simulink model "IP_Core_SS_Switch_and_PWM"  (R2021a)
settings: Solver=VariableStepAuto  StartTime=0.0  StopTime=0.001  RelTol=1e-3
values from neighbouring files (symbols this model uses):
  f_FPGA_clk = 100e6    (= 100000000)    [Init_IP_Core.m]
  T_FPGA_clk = 1/f_FPGA_clk    (= 1e-08)    [Init_IP_Core.m]
libraries: hdlsllib x4, simulink x2
(part 2 of 3)

== system IP_Core_SS_Switch_and_PWM/PWM_and_Switching_Signal_Control/GenPWM/LimitPulseWidth2 ==
  note: Set pulse width in percent
  ref_sig : Inport
  min_pulse_width : Inport  Port=2
  Add : Sum  Inputs=+-  OutDataTypeStr=Inherit: Same as first input
  Constant : Constant  OutDataTypeStr=fixdt(1,18,16)  SampleTime=T_FPGA_clk
  Constant1 : Constant  Value=1.01  OutDataTypeStr=fixdt(1,18,16)  SampleTime=T_FPGA_clk
  Constant2 : Constant  Value=0  OutDataTypeStr=fixdt(1,18,16)  SampleTime=T_FPGA_clk
  Logical Operator : Logic  Operator=OR  AllPortsSameDT=off  OutDataTypeStr=boolean
  Relational Operator : RelationalOperator  Operator=>  OutDataTypeStr=boolean  RndMeth=Nearest
  Relational Operator1 : RelationalOperator  Operator=<  OutDataTypeStr=boolean  RndMeth=Nearest
  Saturation : Saturate  UpperLimit=1  LowerLimit=0  OutDataTypeStr=fixdt(1,18,16)
  Switch1 : Switch  Criteria=u2 > Threshold
  Switch6 : Switch  Criteria=u2 > Threshold
  ref_sig_limit : Outport  VectorParamsAs1DForOutWhenUnconnected=off
  wires:
  Constant/1 -> Add/1
  min_pulse_width/1 -> Add/2, Saturation/1
  Add/1 -> Relational Operator/2
  ref_sig/1 -> Switch6/3, Relational Operator/1, Relational Operator1/1
  Relational Operator/1 -> Logical Operator/1
  Relational Operator1/1 -> Logical Operator/2, Switch1/2
  Logical Operator/1 -> Switch6/2
  Constant1/1 -> Switch1/3
  Switch1/1 -> Switch6/1
  Constant2/1 -> Switch1/1
  Switch6/1 -> ref_sig_limit/1
  Saturation/1 -> Relational Operator1/2

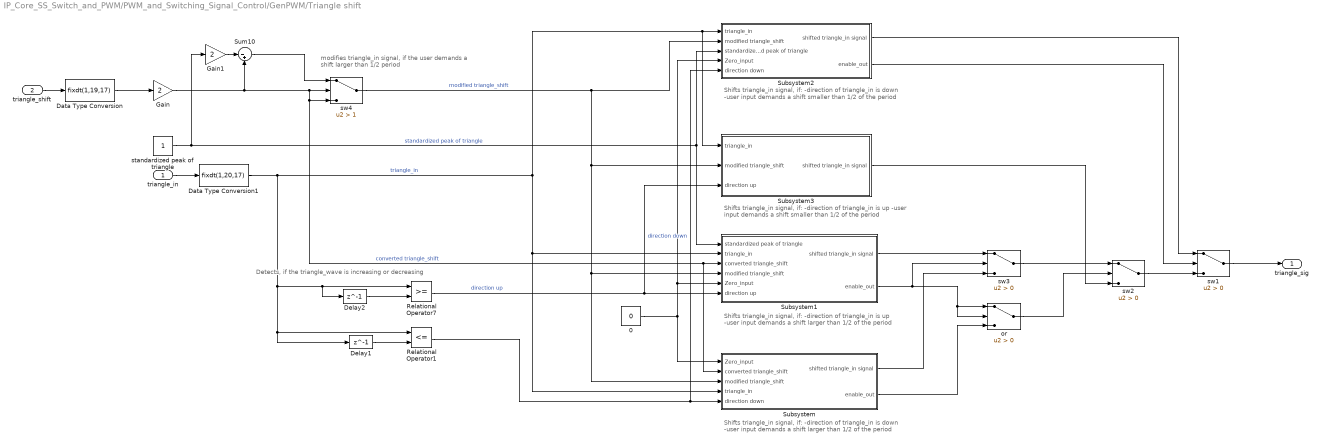
== system IP_Core_SS_Switch_and_PWM/PWM_and_Switching_Signal_Control/GenPWM/Triangle shift ==
  note: modifies triangle_in signal,
      | if the user demands a shift larger than 1/2 period
  note: Detects, if the triangle_wave is increasing or decreasing
  note: Shifts triangle_in signal, if:
      | -direction of triangle_in is down
      | -user input demands a shift larger than 1/2 of the period
  note: Shifts triangle_in signal, if:
      | -direction of triangle_in is up
      | -user input demands a shift larger than 1/2 of the period
  note: Shifts triangle_in signal, if:
      | -direction of triangle_in is up
      | -user input demands a shift smaller than 1/2 of the period
  note: Shifts triangle_in signal, if:
      | -direction of triangle_in is down
      | -user input demands a shift smaller than 1/2 of the period
  triangle_in : Inport
  triangle_shift : Inport  Port=2
  0 : Constant  Value=0  OutDataTypeStr=boolean  SampleTime=T_FPGA_clk
  Data Type Conversion : DataTypeConversion  OutDataTypeStr=fixdt(1,19,17)
  Data Type Conversion1 : DataTypeConversion  OutDataTypeStr=fixdt(1,20,17)
  Delay1 : Delay  DelayLength=1
  Delay2 : Delay  DelayLength=1
  Gain : Gain  Gain=2  OutDataTypeStr=fixdt(1,20,17)
  Gain1 : Gain  Gain=2  OutDataTypeStr=fixdt(1,20,17)
  Relational Operator1 : RelationalOperator  Operator=<=  OutDataTypeStr=boolean  RndMeth=Nearest
  Relational Operator7 : RelationalOperator  OutDataTypeStr=boolean  RndMeth=Nearest
  Subsystem : Subsystem
  Subsystem1 : Subsystem
  Subsystem2 : Subsystem
  Subsystem3 : Subsystem
  Sum10 : Sum  Inputs=|-+  OutDataTypeStr=fixdt(1,20,17)
  or : Switch  Criteria=u2 > Threshold
  standardized peak of triangle : Constant  OutDataTypeStr=fixdt(0,21,17)  SampleTime=T_FPGA_clk
  sw1 : Switch  Criteria=u2 > Threshold  OutDataTypeStr=fixdt(1,18,16)
  sw2 : Switch  Criteria=u2 > Threshold
  sw3 : Switch  Criteria=u2 > Threshold
  sw4 : Switch  Criteria=u2 > Threshold  Threshold=1  OutDataTypeStr=fixdt(1,20,17)
  triangle_sig : Outport  VectorParamsAs1DForOutWhenUnconnected=off
  wires:
  Delay2/1 -> Relational Operator7/2
  Data Type Conversion1/1 -> Subsystem3/1(triangle_in), Subsystem2/1(triangle_in), Subsystem/4(triangle_in), Subsystem1/2(triangle_in), Relational Operator1/1, Delay1/1, Delay2/1, Relational Operator7/1  "triangle_in"
  sw3/1 -> sw2/1
  Relational Operator7/1 -> Subsystem1/6(direction up), Subsystem3/3(direction up)  "direction up"
  or/1 -> sw2/2
  sw4/1 -> Subsystem3/2(modified triangle_shift), Subsystem/3(modified triangle_shift), Subsystem1/4(modified triangle_shift), Subsystem2/2(modified triangle_shift)  "modified triangle_shift"
  Gain/1 -> Sum10/2, Subsystem/2(converted triangle_shift), Subsystem1/3(converted triangle_shift), sw4/3, sw4/2  "converted triangle_shift"
  Sum10/1 -> sw4/1
  sw1/1 -> triangle_sig/1
  standardized peak of triangle/1 -> Subsystem2/3(standardized peak of triangle), Subsystem1/1(standardized peak of triangle), Gain1/1  "standardized peak of triangle"
  triangle_shift/1 -> Data Type Conversion/1
  Gain1/1 -> Sum10/1
  sw2/1 -> sw1/3
  Data Type Conversion/1 -> Gain/1
  triangle_in/1 -> Data Type Conversion1/1
  Relational Operator1/1 -> Subsystem/5(direction down), Subsystem2/5(direction down)  "direction down"
  Delay1/1 -> Relational Operator1/2
  0/1 -> Subsystem2/4(Zero_input), Subsystem1/5(Zero_input), Subsystem/1(Zero_input)
  Subsystem/1(shifted triangle_in signal) -> sw3/3
  Subsystem/2(enable_out) -> or/3
  Subsystem1/2(enable_out) -> or/2, or/1, sw3/2
  Subsystem1/1(shifted triangle_in signal) -> sw3/1
  Subsystem2/1(shifted triangle_in signal) -> sw1/1
  Subsystem2/2(enable_out) -> sw1/2
  Subsystem3/1(shifted triangle_in signal) -> sw2/3

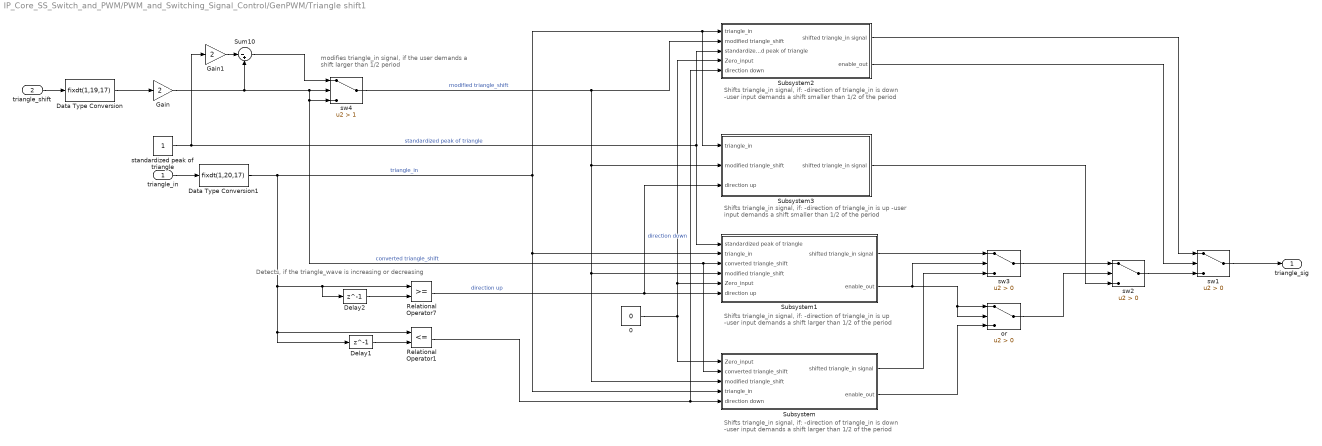
== system IP_Core_SS_Switch_and_PWM/PWM_and_Switching_Signal_Control/GenPWM/Triangle shift1 ==
  note: modifies triangle_in signal,
      | if the user demands a shift larger than 1/2 period
  note: Detects, if the triangle_wave is increasing or decreasing
  note: Shifts triangle_in signal, if:
      | -direction of triangle_in is down
      | -user input demands a shift larger than 1/2 of the period
  note: Shifts triangle_in signal, if:
      | -direction of triangle_in is up
      | -user input demands a shift larger than 1/2 of the period
  note: Shifts triangle_in signal, if:
      | -direction of triangle_in is up
      | -user input demands a shift smaller than 1/2 of the period
  note: Shifts triangle_in signal, if:
      | -direction of triangle_in is down
      | -user input demands a shift smaller than 1/2 of the period
  triangle_in : Inport
  triangle_shift : Inport  Port=2
  0 : Constant  Value=0  OutDataTypeStr=boolean  SampleTime=T_FPGA_clk
  Data Type Conversion : DataTypeConversion  OutDataTypeStr=fixdt(1,19,17)
  Data Type Conversion1 : DataTypeConversion  OutDataTypeStr=fixdt(1,20,17)
  Delay1 : Delay  DelayLength=1
  Delay2 : Delay  DelayLength=1
  Gain : Gain  Gain=2  OutDataTypeStr=fixdt(1,20,17)
  Gain1 : Gain  Gain=2  OutDataTypeStr=fixdt(1,20,17)
  Relational Operator1 : RelationalOperator  Operator=<=  OutDataTypeStr=boolean  RndMeth=Nearest
  Relational Operator7 : RelationalOperator  OutDataTypeStr=boolean  RndMeth=Nearest
  Subsystem : Subsystem
  Subsystem1 : Subsystem
  Subsystem2 : Subsystem
  Subsystem3 : Subsystem
  Sum10 : Sum  Inputs=|-+  OutDataTypeStr=fixdt(1,20,17)
  or : Switch  Criteria=u2 > Threshold
  standardized peak of triangle : Constant  OutDataTypeStr=fixdt(0,21,17)  SampleTime=T_FPGA_clk
  sw1 : Switch  Criteria=u2 > Threshold  OutDataTypeStr=fixdt(1,18,16)
  sw2 : Switch  Criteria=u2 > Threshold
  sw3 : Switch  Criteria=u2 > Threshold
  sw4 : Switch  Criteria=u2 > Threshold  Threshold=1  OutDataTypeStr=fixdt(1,20,17)
  triangle_sig : Outport  VectorParamsAs1DForOutWhenUnconnected=off
  wires:
  Delay2/1 -> Relational Operator7/2
  Data Type Conversion1/1 -> Subsystem3/1(triangle_in), Subsystem2/1(triangle_in), Subsystem/4(triangle_in), Subsystem1/2(triangle_in), Relational Operator1/1, Delay1/1, Delay2/1, Relational Operator7/1  "triangle_in"
  sw3/1 -> sw2/1
  Relational Operator7/1 -> Subsystem1/6(direction up), Subsystem3/3(direction up)  "direction up"
  or/1 -> sw2/2
  sw4/1 -> Subsystem3/2(modified triangle_shift), Subsystem/3(modified triangle_shift), Subsystem1/4(modified triangle_shift), Subsystem2/2(modified triangle_shift)  "modified triangle_shift"
  Gain/1 -> Sum10/2, Subsystem/2(converted triangle_shift), Subsystem1/3(converted triangle_shift), sw4/3, sw4/2  "converted triangle_shift"
  Sum10/1 -> sw4/1
  sw1/1 -> triangle_sig/1
  standardized peak of triangle/1 -> Subsystem2/3(standardized peak of triangle), Subsystem1/1(standardized peak of triangle), Gain1/1  "standardized peak of triangle"
  triangle_shift/1 -> Data Type Conversion/1
  Gain1/1 -> Sum10/1
  sw2/1 -> sw1/3
  Data Type Conversion/1 -> Gain/1
  triangle_in/1 -> Data Type Conversion1/1
  Relational Operator1/1 -> Subsystem/5(direction down), Subsystem2/5(direction down)  "direction down"
  Delay1/1 -> Relational Operator1/2
  0/1 -> Subsystem2/4(Zero_input), Subsystem1/5(Zero_input), Subsystem/1(Zero_input)
  Subsystem/1(shifted triangle_in signal) -> sw3/3
  Subsystem/2(enable_out) -> or/3
  Subsystem1/2(enable_out) -> or/2, or/1, sw3/2
  Subsystem1/1(shifted triangle_in signal) -> sw3/1
  Subsystem2/1(shifted triangle_in signal) -> sw1/1
  Subsystem2/2(enable_out) -> sw1/2
  Subsystem3/1(shifted triangle_in signal) -> sw2/3

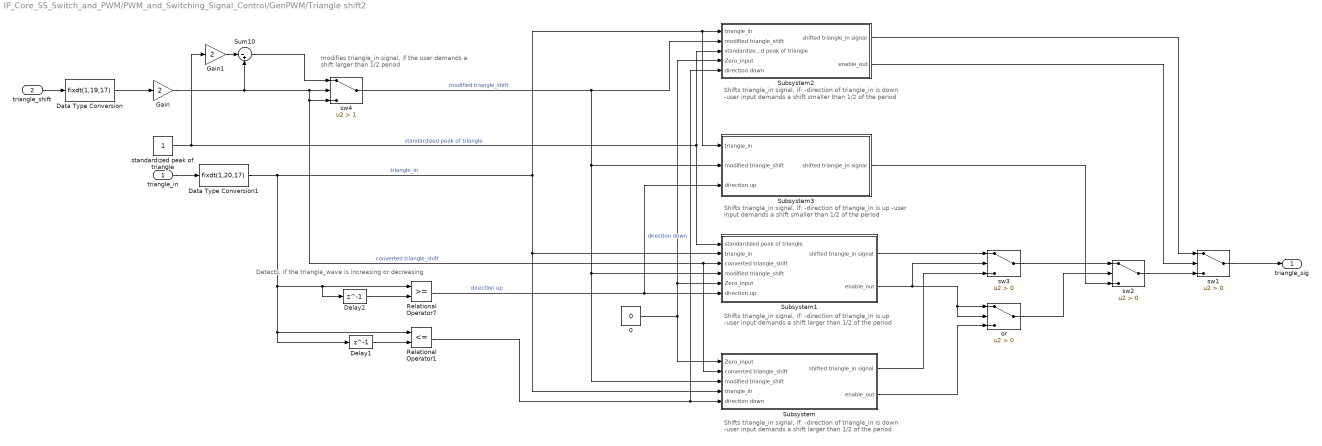
== system IP_Core_SS_Switch_and_PWM/PWM_and_Switching_Signal_Control/GenPWM/Triangle shift2 ==
  note: modifies triangle_in signal,
      | if the user demands a shift larger than 1/2 period
  note: Detects, if the triangle_wave is increasing or decreasing
  note: Shifts triangle_in signal, if:
      | -direction of triangle_in is down
      | -user input demands a shift larger than 1/2 of the period
  note: Shifts triangle_in signal, if:
      | -direction of triangle_in is up
      | -user input demands a shift larger than 1/2 of the period
  note: Shifts triangle_in signal, if:
      | -direction of triangle_in is up
      | -user input demands a shift smaller than 1/2 of the period
  note: Shifts triangle_in signal, if:
      | -direction of triangle_in is down
      | -user input demands a shift smaller than 1/2 of the period
  triangle_in : Inport
  triangle_shift : Inport  Port=2
  0 : Constant  Value=0  OutDataTypeStr=boolean  SampleTime=T_FPGA_clk
  Data Type Conversion : DataTypeConversion  OutDataTypeStr=fixdt(1,19,17)
  Data Type Conversion1 : DataTypeConversion  OutDataTypeStr=fixdt(1,20,17)
  Delay1 : Delay  DelayLength=1
  Delay2 : Delay  DelayLength=1
  Gain : Gain  Gain=2  OutDataTypeStr=fixdt(1,20,17)
  Gain1 : Gain  Gain=2  OutDataTypeStr=fixdt(1,20,17)
  Relational Operator1 : RelationalOperator  Operator=<=  OutDataTypeStr=boolean  RndMeth=Nearest
  Relational Operator7 : RelationalOperator  OutDataTypeStr=boolean  RndMeth=Nearest
  Subsystem : Subsystem
  Subsystem1 : Subsystem
  Subsystem2 : Subsystem
  Subsystem3 : Subsystem
  Sum10 : Sum  Inputs=|-+  OutDataTypeStr=fixdt(1,20,17)
  or : Switch  Criteria=u2 > Threshold
  standardized peak of triangle : Constant  OutDataTypeStr=fixdt(0,21,17)  SampleTime=T_FPGA_clk
  sw1 : Switch  Criteria=u2 > Threshold  OutDataTypeStr=fixdt(1,18,16)
  sw2 : Switch  Criteria=u2 > Threshold
  sw3 : Switch  Criteria=u2 > Threshold
  sw4 : Switch  Criteria=u2 > Threshold  Threshold=1  OutDataTypeStr=fixdt(1,20,17)
  triangle_sig : Outport  VectorParamsAs1DForOutWhenUnconnected=off
  wires:
  Delay2/1 -> Relational Operator7/2
  Data Type Conversion1/1 -> Subsystem3/1(triangle_in), Subsystem2/1(triangle_in), Subsystem/4(triangle_in), Subsystem1/2(triangle_in), Relational Operator1/1, Delay1/1, Delay2/1, Relational Operator7/1  "triangle_in"
  sw3/1 -> sw2/1
  Relational Operator7/1 -> Subsystem1/6(direction up), Subsystem3/3(direction up)  "direction up"
  or/1 -> sw2/2
  sw4/1 -> Subsystem3/2(modified triangle_shift), Subsystem/3(modified triangle_shift), Subsystem1/4(modified triangle_shift), Subsystem2/2(modified triangle_shift)  "modified triangle_shift"
  Gain/1 -> Sum10/2, Subsystem/2(converted triangle_shift), Subsystem1/3(converted triangle_shift), sw4/3, sw4/2  "converted triangle_shift"
  Sum10/1 -> sw4/1
  sw1/1 -> triangle_sig/1
  standardized peak of triangle/1 -> Subsystem2/3(standardized peak of triangle), Subsystem1/1(standardized peak of triangle), Gain1/1  "standardized peak of triangle"
  triangle_shift/1 -> Data Type Conversion/1
  Gain1/1 -> Sum10/1
  sw2/1 -> sw1/3
  Data Type Conversion/1 -> Gain/1
  triangle_in/1 -> Data Type Conversion1/1
  Relational Operator1/1 -> Subsystem/5(direction down), Subsystem2/5(direction down)  "direction down"
  Delay1/1 -> Relational Operator1/2
  0/1 -> Subsystem2/4(Zero_input), Subsystem1/5(Zero_input), Subsystem/1(Zero_input)
  Subsystem/1(shifted triangle_in signal) -> sw3/3
  Subsystem/2(enable_out) -> or/3
  Subsystem1/2(enable_out) -> or/2, or/1, sw3/2
  Subsystem1/1(shifted triangle_in signal) -> sw3/1
  Subsystem2/1(shifted triangle_in signal) -> sw1/1
  Subsystem2/2(enable_out) -> sw1/2
  Subsystem3/1(shifted triangle_in signal) -> sw2/3

== system IP_Core_SS_Switch_and_PWM/PWM_and_Switching_Signal_Control1/GenPWM/Counter Ctrl ==
  note: if (hdl_cnt >= step_cnt)
      | 	dir_ctrl = true;
      | else if (hdl_cnt <= 0)
      | 	dir_ctrl = false;
      | else
      | 	dir_ctrl = dir_ctrl;
  note: scaling triangle amplitude to 100
  hdl_cnt : Inport
  f_carrier_kHz : Inport  Port=2
  T_carrier_us : Inport  Port=3
  Constant1 : Constant  Value=0  OutDataTypeStr=fixdt(0,20,0)  SampleTime=T_FPGA_clk
  Constant11 : Constant  Value=0  OutDataTypeStr=fixdt(0,20,0)  SampleTime=T_FPGA_clk
  Constant12 : Constant  Value=false  SampleTime=T_FPGA_clk
  Constant14 : Constant  Value=true  SampleTime=T_FPGA_clk
  Delay : Delay  DelayLength=1
  Delay6 : Delay  DelayLength=1
  Logical Operator : Logic  Operator=OR  AllPortsSameDT=off  OutDataTypeStr=boolean
  Product : Product  OutDataTypeStr=fixdt(0,18,17)
  Relational Operator1 : RelationalOperator  Operator===  OutDataTypeStr=boolean  RndMeth=Nearest
  Relational Operator2 : RelationalOperator  Operator===  OutDataTypeStr=boolean  RndMeth=Nearest
  Relational Operator4 : RelationalOperator  OutDataTypeStr=boolean  RndMeth=Nearest
  Relational Operator5 : RelationalOperator  Operator=<=  OutDataTypeStr=boolean  RndMeth=Nearest
  Scope9 : Scope  NumInputPorts=2
  Switch6 : Switch  Criteria=u2 > Threshold
  Switch7 : Switch  Criteria=u2 > Threshold
  dir_ctrl : Outport  VectorParamsAs1DForOutWhenUnconnected=off
  triangle_sig : Outport  Port=2  VectorParamsAs1DForOutWhenUnconnected=off
  Period_CenterMax : Outport  Port=3  VectorParamsAs1DForOutWhenUnconnected=off
  Period_CenterMin : Outport  Port=4  VectorParamsAs1DForOutWhenUnconnected=off
  wires:
  hdl_cnt/1 -> Relational Operator2/1, Relational Operator1/1, Relational Operator5/1, Relational Operator4/1, Product/1, Scope9/1
  Switch6/1 -> Delay6/1, dir_ctrl/1
  Relational Operator4/1 -> Switch7/2, Logical Operator/1
  Relational Operator5/1 -> Logical Operator/2
  Constant11/1 -> Relational Operator5/2
  Logical Operator/1 -> Switch6/2
  Switch7/1 -> Switch6/1
  Constant12/1 -> Switch7/1
  Constant14/1 -> Switch7/3
  Delay6/1 -> Switch6/3
  T_carrier_us/1 -> Relational Operator4/2, Relational Operator1/2
  f_carrier_kHz/1 -> Delay/1
  Delay/1 -> Scope9/2, Product/2
  Relational Operator1/1 -> Period_CenterMax/1
  Relational Operator2/1 -> Period_CenterMin/1
  Constant1/1 -> Relational Operator2/2
  Product/1 -> triangle_sig/1

== system IP_Core_SS_Switch_and_PWM/PWM_and_Switching_Signal_Control1/GenPWM/LimitPulseWidth ==
  note: Set pulse width between 0-1
  ref_sig : Inport
  min_pulse_width : Inport  Port=2
  Add : Sum  Inputs=+-  OutDataTypeStr=Inherit: Same as first input
  Constant : Constant  OutDataTypeStr=fixdt(1,18,16)  SampleTime=T_FPGA_clk
  Constant1 : Constant  Value=1.01  OutDataTypeStr=fixdt(1,18,16)  SampleTime=T_FPGA_clk
  Constant2 : Constant  Value=0  OutDataTypeStr=fixdt(1,18,16)  SampleTime=T_FPGA_clk
  Logical Operator : Logic  Operator=OR  AllPortsSameDT=off  OutDataTypeStr=boolean
  Relational Operator : RelationalOperator  Operator=>  OutDataTypeStr=boolean  RndMeth=Nearest
  Relational Operator1 : RelationalOperator  Operator=<  OutDataTypeStr=boolean  RndMeth=Nearest
  Saturation : Saturate  UpperLimit=1  LowerLimit=0  OutDataTypeStr=fixdt(1,18,16)
  Switch1 : Switch  Criteria=u2 > Threshold
  Switch6 : Switch  Criteria=u2 > Threshold
  ref_sig_limit : Outport  VectorParamsAs1DForOutWhenUnconnected=off
  wires:
  Constant/1 -> Add/1
  min_pulse_width/1 -> Add/2, Saturation/1
  Add/1 -> Relational Operator/2
  ref_sig/1 -> Switch6/3, Relational Operator/1, Relational Operator1/1
  Relational Operator/1 -> Logical Operator/1
  Relational Operator1/1 -> Logical Operator/2, Switch1/2
  Logical Operator/1 -> Switch6/2
  Constant1/1 -> Switch1/3
  Switch1/1 -> Switch6/1
  Constant2/1 -> Switch1/1
  Switch6/1 -> ref_sig_limit/1
  Saturation/1 -> Relational Operator1/2

== system IP_Core_SS_Switch_and_PWM/PWM_and_Switching_Signal_Control1/GenPWM/LimitPulseWidth1 ==
  note: Set pulse width in percent
  ref_sig : Inport
  min_pulse_width : Inport  Port=2
  Add : Sum  Inputs=+-  OutDataTypeStr=Inherit: Same as first input
  Constant : Constant  OutDataTypeStr=fixdt(1,18,16)  SampleTime=T_FPGA_clk
  Constant1 : Constant  Value=1.01  OutDataTypeStr=fixdt(1,18,16)  SampleTime=T_FPGA_clk
  Constant2 : Constant  Value=0  OutDataTypeStr=fixdt(1,18,16)  SampleTime=T_FPGA_clk
  Logical Operator : Logic  Operator=OR  AllPortsSameDT=off  OutDataTypeStr=boolean
  Relational Operator : RelationalOperator  Operator=>  OutDataTypeStr=boolean  RndMeth=Nearest
  Relational Operator1 : RelationalOperator  Operator=<  OutDataTypeStr=boolean  RndMeth=Nearest
  Saturation : Saturate  UpperLimit=1  LowerLimit=0  OutDataTypeStr=fixdt(1,18,16)
  Switch1 : Switch  Criteria=u2 > Threshold
  Switch6 : Switch  Criteria=u2 > Threshold
  ref_sig_limit : Outport  VectorParamsAs1DForOutWhenUnconnected=off
  wires:
  Constant/1 -> Add/1
  min_pulse_width/1 -> Add/2, Saturation/1
  Add/1 -> Relational Operator/2
  ref_sig/1 -> Switch6/3, Relational Operator/1, Relational Operator1/1
  Relational Operator/1 -> Logical Operator/1
  Relational Operator1/1 -> Logical Operator/2, Switch1/2
  Logical Operator/1 -> Switch6/2
  Constant1/1 -> Switch1/3
  Switch1/1 -> Switch6/1
  Constant2/1 -> Switch1/1
  Switch6/1 -> ref_sig_limit/1
  Saturation/1 -> Relational Operator1/2

== system IP_Core_SS_Switch_and_PWM/PWM_and_Switching_Signal_Control1/GenPWM/LimitPulseWidth2 ==
  note: Set pulse width in percent
  ref_sig : Inport
  min_pulse_width : Inport  Port=2
  Add : Sum  Inputs=+-  OutDataTypeStr=Inherit: Same as first input
  Constant : Constant  OutDataTypeStr=fixdt(1,18,16)  SampleTime=T_FPGA_clk
  Constant1 : Constant  Value=1.01  OutDataTypeStr=fixdt(1,18,16)  SampleTime=T_FPGA_clk
  Constant2 : Constant  Value=0  OutDataTypeStr=fixdt(1,18,16)  SampleTime=T_FPGA_clk
  Logical Operator : Logic  Operator=OR  AllPortsSameDT=off  OutDataTypeStr=boolean
  Relational Operator : RelationalOperator  Operator=>  OutDataTypeStr=boolean  RndMeth=Nearest
  Relational Operator1 : RelationalOperator  Operator=<  OutDataTypeStr=boolean  RndMeth=Nearest
  Saturation : Saturate  UpperLimit=1  LowerLimit=0  OutDataTypeStr=fixdt(1,18,16)
  Switch1 : Switch  Criteria=u2 > Threshold
  Switch6 : Switch  Criteria=u2 > Threshold
  ref_sig_limit : Outport  VectorParamsAs1DForOutWhenUnconnected=off
  wires:
  Constant/1 -> Add/1
  min_pulse_width/1 -> Add/2, Saturation/1
  Add/1 -> Relational Operator/2
  ref_sig/1 -> Switch6/3, Relational Operator/1, Relational Operator1/1
  Relational Operator/1 -> Logical Operator/1
  Relational Operator1/1 -> Logical Operator/2, Switch1/2
  Logical Operator/1 -> Switch6/2
  Constant1/1 -> Switch1/3
  Switch1/1 -> Switch6/1
  Constant2/1 -> Switch1/1
  Switch6/1 -> ref_sig_limit/1
  Saturation/1 -> Relational Operator1/2

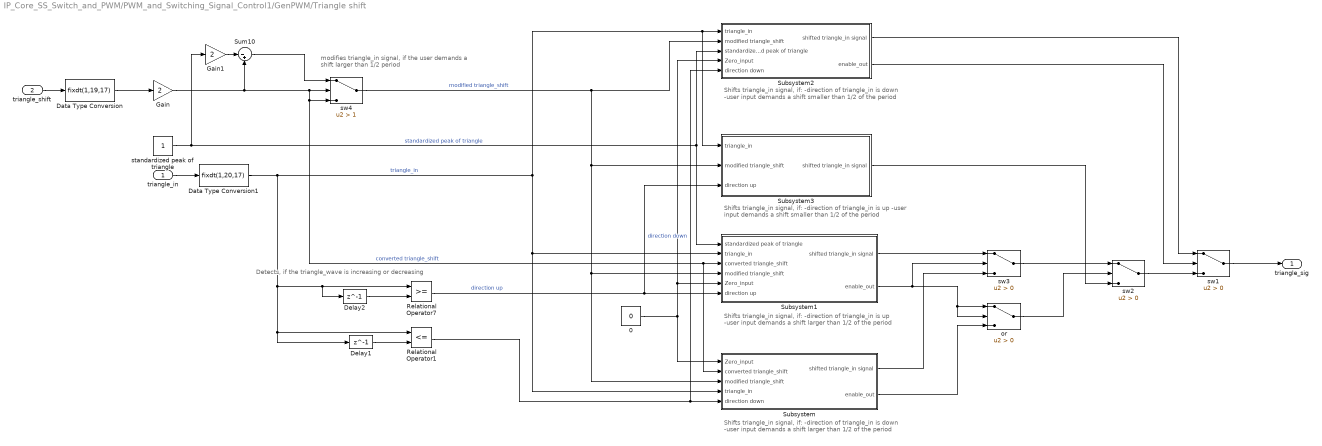
== system IP_Core_SS_Switch_and_PWM/PWM_and_Switching_Signal_Control1/GenPWM/Triangle shift ==
  note: modifies triangle_in signal,
      | if the user demands a shift larger than 1/2 period
  note: Detects, if the triangle_wave is increasing or decreasing
  note: Shifts triangle_in signal, if:
      | -direction of triangle_in is down
      | -user input demands a shift larger than 1/2 of the period
  note: Shifts triangle_in signal, if:
      | -direction of triangle_in is up
      | -user input demands a shift larger than 1/2 of the period
  note: Shifts triangle_in signal, if:
      | -direction of triangle_in is up
      | -user input demands a shift smaller than 1/2 of the period
  note: Shifts triangle_in signal, if:
      | -direction of triangle_in is down
      | -user input demands a shift smaller than 1/2 of the period
  triangle_in : Inport
  triangle_shift : Inport  Port=2
  0 : Constant  Value=0  OutDataTypeStr=boolean  SampleTime=T_FPGA_clk
  Data Type Conversion : DataTypeConversion  OutDataTypeStr=fixdt(1,19,17)
  Data Type Conversion1 : DataTypeConversion  OutDataTypeStr=fixdt(1,20,17)
  Delay1 : Delay  DelayLength=1
  Delay2 : Delay  DelayLength=1
  Gain : Gain  Gain=2  OutDataTypeStr=fixdt(1,20,17)
  Gain1 : Gain  Gain=2  OutDataTypeStr=fixdt(1,20,17)
  Relational Operator1 : RelationalOperator  Operator=<=  OutDataTypeStr=boolean  RndMeth=Nearest
  Relational Operator7 : RelationalOperator  OutDataTypeStr=boolean  RndMeth=Nearest
  Subsystem : Subsystem
  Subsystem1 : Subsystem
  Subsystem2 : Subsystem
  Subsystem3 : Subsystem
  Sum10 : Sum  Inputs=|-+  OutDataTypeStr=fixdt(1,20,17)
  or : Switch  Criteria=u2 > Threshold
  standardized peak of triangle : Constant  OutDataTypeStr=fixdt(0,21,17)  SampleTime=T_FPGA_clk
  sw1 : Switch  Criteria=u2 > Threshold  OutDataTypeStr=fixdt(1,18,16)
  sw2 : Switch  Criteria=u2 > Threshold
  sw3 : Switch  Criteria=u2 > Threshold
  sw4 : Switch  Criteria=u2 > Threshold  Threshold=1  OutDataTypeStr=fixdt(1,20,17)
  triangle_sig : Outport  VectorParamsAs1DForOutWhenUnconnected=off
  wires:
  Delay2/1 -> Relational Operator7/2
  Data Type Conversion1/1 -> Subsystem3/1(triangle_in), Subsystem2/1(triangle_in), Subsystem/4(triangle_in), Subsystem1/2(triangle_in), Relational Operator1/1, Delay1/1, Delay2/1, Relational Operator7/1  "triangle_in"
  sw3/1 -> sw2/1
  Relational Operator7/1 -> Subsystem1/6(direction up), Subsystem3/3(direction up)  "direction up"
  or/1 -> sw2/2
  sw4/1 -> Subsystem3/2(modified triangle_shift), Subsystem/3(modified triangle_shift), Subsystem1/4(modified triangle_shift), Subsystem2/2(modified triangle_shift)  "modified triangle_shift"
  Gain/1 -> Sum10/2, Subsystem/2(converted triangle_shift), Subsystem1/3(converted triangle_shift), sw4/3, sw4/2  "converted triangle_shift"
  Sum10/1 -> sw4/1
  sw1/1 -> triangle_sig/1
  standardized peak of triangle/1 -> Subsystem2/3(standardized peak of triangle), Subsystem1/1(standardized peak of triangle), Gain1/1  "standardized peak of triangle"
  triangle_shift/1 -> Data Type Conversion/1
  Gain1/1 -> Sum10/1
  sw2/1 -> sw1/3
  Data Type Conversion/1 -> Gain/1
  triangle_in/1 -> Data Type Conversion1/1
  Relational Operator1/1 -> Subsystem/5(direction down), Subsystem2/5(direction down)  "direction down"
  Delay1/1 -> Relational Operator1/2
  0/1 -> Subsystem2/4(Zero_input), Subsystem1/5(Zero_input), Subsystem/1(Zero_input)
  Subsystem/1(shifted triangle_in signal) -> sw3/3
  Subsystem/2(enable_out) -> or/3
  Subsystem1/2(enable_out) -> or/2, or/1, sw3/2
  Subsystem1/1(shifted triangle_in signal) -> sw3/1
  Subsystem2/1(shifted triangle_in signal) -> sw1/1
  Subsystem2/2(enable_out) -> sw1/2
  Subsystem3/1(shifted triangle_in signal) -> sw2/3

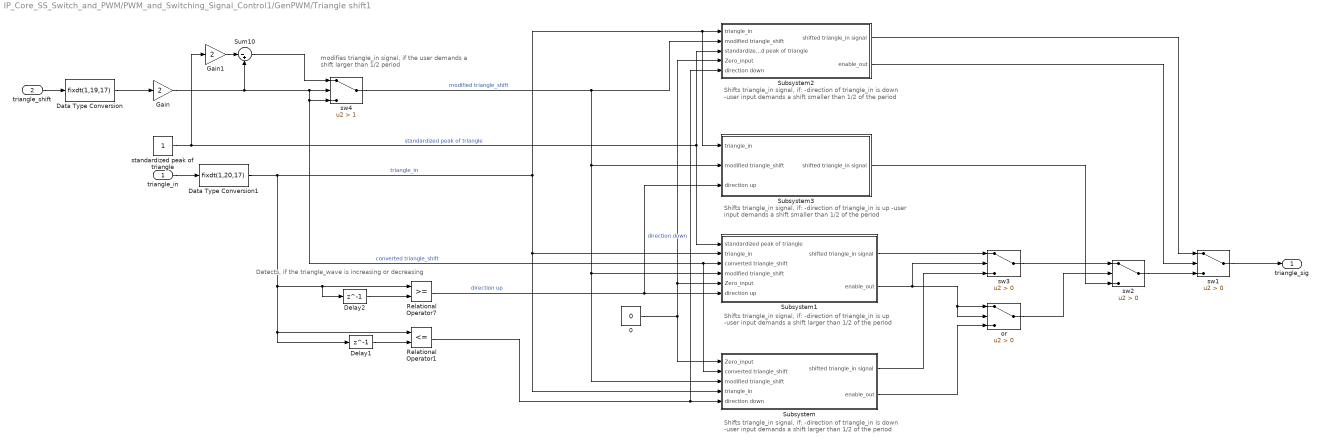
== system IP_Core_SS_Switch_and_PWM/PWM_and_Switching_Signal_Control1/GenPWM/Triangle shift1 ==
  note: modifies triangle_in signal,
      | if the user demands a shift larger than 1/2 period
  note: Detects, if the triangle_wave is increasing or decreasing
  note: Shifts triangle_in signal, if:
      | -direction of triangle_in is down
      | -user input demands a shift larger than 1/2 of the period
  note: Shifts triangle_in signal, if:
      | -direction of triangle_in is up
      | -user input demands a shift larger than 1/2 of the period
  note: Shifts triangle_in signal, if:
      | -direction of triangle_in is up
      | -user input demands a shift smaller than 1/2 of the period
  note: Shifts triangle_in signal, if:
      | -direction of triangle_in is down
      | -user input demands a shift smaller than 1/2 of the period
  triangle_in : Inport
  triangle_shift : Inport  Port=2
  0 : Constant  Value=0  OutDataTypeStr=boolean  SampleTime=T_FPGA_clk
  Data Type Conversion : DataTypeConversion  OutDataTypeStr=fixdt(1,19,17)
  Data Type Conversion1 : DataTypeConversion  OutDataTypeStr=fixdt(1,20,17)
  Delay1 : Delay  DelayLength=1
  Delay2 : Delay  DelayLength=1
  Gain : Gain  Gain=2  OutDataTypeStr=fixdt(1,20,17)
  Gain1 : Gain  Gain=2  OutDataTypeStr=fixdt(1,20,17)
  Relational Operator1 : RelationalOperator  Operator=<=  OutDataTypeStr=boolean  RndMeth=Nearest
  Relational Operator7 : RelationalOperator  OutDataTypeStr=boolean  RndMeth=Nearest
  Subsystem : Subsystem
  Subsystem1 : Subsystem
  Subsystem2 : Subsystem
  Subsystem3 : Subsystem
  Sum10 : Sum  Inputs=|-+  OutDataTypeStr=fixdt(1,20,17)
  or : Switch  Criteria=u2 > Threshold
  standardized peak of triangle : Constant  OutDataTypeStr=fixdt(0,21,17)  SampleTime=T_FPGA_clk
  sw1 : Switch  Criteria=u2 > Threshold  OutDataTypeStr=fixdt(1,18,16)
  sw2 : Switch  Criteria=u2 > Threshold
  sw3 : Switch  Criteria=u2 > Threshold
  sw4 : Switch  Criteria=u2 > Threshold  Threshold=1  OutDataTypeStr=fixdt(1,20,17)
  triangle_sig : Outport  VectorParamsAs1DForOutWhenUnconnected=off
  wires:
  Delay2/1 -> Relational Operator7/2
  Data Type Conversion1/1 -> Subsystem3/1(triangle_in), Subsystem2/1(triangle_in), Subsystem/4(triangle_in), Subsystem1/2(triangle_in), Relational Operator1/1, Delay1/1, Delay2/1, Relational Operator7/1  "triangle_in"
  sw3/1 -> sw2/1
  Relational Operator7/1 -> Subsystem1/6(direction up), Subsystem3/3(direction up)  "direction up"
  or/1 -> sw2/2
  sw4/1 -> Subsystem3/2(modified triangle_shift), Subsystem/3(modified triangle_shift), Subsystem1/4(modified triangle_shift), Subsystem2/2(modified triangle_shift)  "modified triangle_shift"
  Gain/1 -> Sum10/2, Subsystem/2(converted triangle_shift), Subsystem1/3(converted triangle_shift), sw4/3, sw4/2  "converted triangle_shift"
  Sum10/1 -> sw4/1
  sw1/1 -> triangle_sig/1
  standardized peak of triangle/1 -> Subsystem2/3(standardized peak of triangle), Subsystem1/1(standardized peak of triangle), Gain1/1  "standardized peak of triangle"
  triangle_shift/1 -> Data Type Conversion/1
  Gain1/1 -> Sum10/1
  sw2/1 -> sw1/3
  Data Type Conversion/1 -> Gain/1
  triangle_in/1 -> Data Type Conversion1/1
  Relational Operator1/1 -> Subsystem/5(direction down), Subsystem2/5(direction down)  "direction down"
  Delay1/1 -> Relational Operator1/2
  0/1 -> Subsystem2/4(Zero_input), Subsystem1/5(Zero_input), Subsystem/1(Zero_input)
  Subsystem/1(shifted triangle_in signal) -> sw3/3
  Subsystem/2(enable_out) -> or/3
  Subsystem1/2(enable_out) -> or/2, or/1, sw3/2
  Subsystem1/1(shifted triangle_in signal) -> sw3/1
  Subsystem2/1(shifted triangle_in signal) -> sw1/1
  Subsystem2/2(enable_out) -> sw1/2
  Subsystem3/1(shifted triangle_in signal) -> sw2/3

== system IP_Core_SS_Switch_and_PWM/PWM_and_Switching_Signal_Control1/GenPWM/Triangle shift2 ==
  note: modifies triangle_in signal,
      | if the user demands a shift larger than 1/2 period
  note: Detects, if the triangle_wave is increasing or decreasing
  note: Shifts triangle_in signal, if:
      | -direction of triangle_in is down
      | -user input demands a shift larger than 1/2 of the period
  note: Shifts triangle_in signal, if:
      | -direction of triangle_in is up
      | -user input demands a shift larger than 1/2 of the period
  note: Shifts triangle_in signal, if:
      | -direction of triangle_in is up
      | -user input demands a shift smaller than 1/2 of the period
  note: Shifts triangle_in signal, if:
      | -direction of triangle_in is down
      | -user input demands a shift smaller than 1/2 of the period
  triangle_in : Inport
  triangle_shift : Inport  Port=2
  0 : Constant  Value=0  OutDataTypeStr=boolean  SampleTime=T_FPGA_clk
  Data Type Conversion : DataTypeConversion  OutDataTypeStr=fixdt(1,19,17)
  Data Type Conversion1 : DataTypeConversion  OutDataTypeStr=fixdt(1,20,17)
  Delay1 : Delay  DelayLength=1
  Delay2 : Delay  DelayLength=1
  Gain : Gain  Gain=2  OutDataTypeStr=fixdt(1,20,17)
  Gain1 : Gain  Gain=2  OutDataTypeStr=fixdt(1,20,17)
  Relational Operator1 : RelationalOperator  Operator=<=  OutDataTypeStr=boolean  RndMeth=Nearest
  Relational Operator7 : RelationalOperator  OutDataTypeStr=boolean  RndMeth=Nearest
  Subsystem : Subsystem
  Subsystem1 : Subsystem
  Subsystem2 : Subsystem
  Subsystem3 : Subsystem
  Sum10 : Sum  Inputs=|-+  OutDataTypeStr=fixdt(1,20,17)
  or : Switch  Criteria=u2 > Threshold
  standardized peak of triangle : Constant  OutDataTypeStr=fixdt(0,21,17)  SampleTime=T_FPGA_clk
  sw1 : Switch  Criteria=u2 > Threshold  OutDataTypeStr=fixdt(1,18,16)
  sw2 : Switch  Criteria=u2 > Threshold
  sw3 : Switch  Criteria=u2 > Threshold
  sw4 : Switch  Criteria=u2 > Threshold  Threshold=1  OutDataTypeStr=fixdt(1,20,17)
  triangle_sig : Outport  VectorParamsAs1DForOutWhenUnconnected=off
  wires:
  Delay2/1 -> Relational Operator7/2
  Data Type Conversion1/1 -> Subsystem3/1(triangle_in), Subsystem2/1(triangle_in), Subsystem/4(triangle_in), Subsystem1/2(triangle_in), Relational Operator1/1, Delay1/1, Delay2/1, Relational Operator7/1  "triangle_in"
  sw3/1 -> sw2/1
  Relational Operator7/1 -> Subsystem1/6(direction up), Subsystem3/3(direction up)  "direction up"
  or/1 -> sw2/2
  sw4/1 -> Subsystem3/2(modified triangle_shift), Subsystem/3(modified triangle_shift), Subsystem1/4(modified triangle_shift), Subsystem2/2(modified triangle_shift)  "modified triangle_shift"
  Gain/1 -> Sum10/2, Subsystem/2(converted triangle_shift), Subsystem1/3(converted triangle_shift), sw4/3, sw4/2  "converted triangle_shift"
  Sum10/1 -> sw4/1
  sw1/1 -> triangle_sig/1
  standardized peak of triangle/1 -> Subsystem2/3(standardized peak of triangle), Subsystem1/1(standardized peak of triangle), Gain1/1  "standardized peak of triangle"
  triangle_shift/1 -> Data Type Conversion/1
  Gain1/1 -> Sum10/1
  sw2/1 -> sw1/3
  Data Type Conversion/1 -> Gain/1
  triangle_in/1 -> Data Type Conversion1/1
  Relational Operator1/1 -> Subsystem/5(direction down), Subsystem2/5(direction down)  "direction down"
  Delay1/1 -> Relational Operator1/2
  0/1 -> Subsystem2/4(Zero_input), Subsystem1/5(Zero_input), Subsystem/1(Zero_input)
  Subsystem/1(shifted triangle_in signal) -> sw3/3
  Subsystem/2(enable_out) -> or/3
  Subsystem1/2(enable_out) -> or/2, or/1, sw3/2
  Subsystem1/1(shifted triangle_in signal) -> sw3/1
  Subsystem2/1(shifted triangle_in signal) -> sw1/1
  Subsystem2/2(enable_out) -> sw1/2
  Subsystem3/1(shifted triangle_in signal) -> sw2/3

== system IP_Core_SS_Switch_and_PWM/PWM_and_Switching_Signal_Control/GenPWM/Triangle shift/Subsystem ==
  note: AND block replaced with
      | switches for better performance
  Zero_input : Inport
  converted triangle_shift : Inport  Port=2
  modified triangle_shift : Inport  Port=3
  triangle_in : Inport  Port=4
  direction down : Inport  Port=5
  Relational Operator11 : RelationalOperator  Operator=<=  OutDataTypeStr=boolean  RndMeth=Nearest
  Sum8 : Sum  Inputs=|-+
  Unary Minus : UnaryMinus
  and2_1 : Switch  Criteria=u2 > Threshold
  and2_2 : Switch  Criteria=u2 > Threshold
  shifted triangle_in signal : Outport
  enable_out : Outport  Port=2
  wires:
  direction down/1 -> and2_2/2
  Zero_input/1 -> and2_1/3, and2_2/3
  Relational Operator11/1 -> and2_1/2
  and2_1/1 -> and2_2/1
  Sum8/1 -> shifted triangle_in signal/1
  Unary Minus/1 -> Sum8/2, Relational Operator11/2
  triangle_in/1 -> Sum8/1, Relational Operator11/1
  converted triangle_shift/1 -> and2_1/1
  and2_2/1 -> enable_out/1
  modified triangle_shift/1 -> Unary Minus/1

== system IP_Core_SS_Switch_and_PWM/PWM_and_Switching_Signal_Control/GenPWM/Triangle shift/Subsystem1 ==
  note: AND block replaced with
      | switches for better performance
  note: AND block replaced with
      | switches for better performance
  standardized peak of triangle : Inport
  triangle_in : Inport  Port=2
  converted triangle_shift : Inport  Port=3
  modified triangle_shift : Inport  Port=4
  Zero_input : Inport  Port=5
  direction up : Inport  Port=6
  Relational Operator2 : RelationalOperator  OutDataTypeStr=boolean  RndMeth=Nearest
  Sum11 : Sum  Inputs=++-  OutDataTypeStr=fixdt(1,21,17)
  Sum6 : Sum  Inputs=++|
  and1_1 : Switch  Criteria=u2 > Threshold
  and1_2 : Switch  Criteria=u2 > Threshold
  shifted triangle_in signal : Outport
  enable_out : Outport  Port=2
  wires:
  Sum11/1 -> shifted triangle_in signal/1
  Sum6/1 -> Relational Operator2/2, Sum11/2
  and1_1/1 -> and1_2/1
  Relational Operator2/1 -> and1_1/2
  Zero_input/1 -> and1_2/3, and1_1/3
  standardized peak of triangle/1 -> Sum6/2, Sum11/1
  and1_2/1 -> enable_out/1
  converted triangle_shift/1 -> and1_1/1
  direction up/1 -> and1_2/2
  triangle_in/1 -> Relational Operator2/1, Sum11/3
  modified triangle_shift/1 -> Sum6/1

== system IP_Core_SS_Switch_and_PWM/PWM_and_Switching_Signal_Control/GenPWM/Triangle shift/Subsystem2 ==
  triangle_in : Inport
  modified triangle_shift : Inport  Port=2
  standardized peak of triangle : Inport  Port=3
  Zero_input : Inport  Port=4
  direction down : Inport  Port=5
  Relational Operator9 : RelationalOperator  OutDataTypeStr=boolean  RndMeth=Nearest
  Sum1 : Sum  Inputs=|-+
  Sum5 : Sum  Inputs=++-  OutDataTypeStr=fixdt(1,21,17)
  and : Switch  Criteria=u2 > Threshold
  shifted triangle_in signal : Outport
  enable_out : Outport  Port=2
  wires:
  standardized peak of triangle/1 -> Sum1/2, Sum5/2
  Zero_input/1 -> and/3
  Sum1/1 -> Relational Operator9/2, Sum5/1
  Relational Operator9/1 -> and/1
  direction down/1 -> and/2
  and/1 -> enable_out/1
  triangle_in/1 -> Relational Operator9/1, Sum5/3
  Sum5/1 -> shifted triangle_in signal/1
  modified triangle_shift/1 -> Sum1/1

== system IP_Core_SS_Switch_and_PWM/PWM_and_Switching_Signal_Control/GenPWM/Triangle shift/Subsystem3 ==
  triangle_in : Inport
  modified triangle_shift : Inport  Port=2
  direction up : Inport  Port=3
  Relational Operator6 : RelationalOperator  Operator=<=  OutDataTypeStr=boolean  RndMeth=Nearest
  Sum2 : Sum  Inputs=|-+
  Sum3 : Sum  Inputs=|+-
  Sum4 : Sum  Inputs=|++
  Switch3 : Switch  Criteria=u2 > Threshold
  sw : Switch  Criteria=u2 > Threshold
  shifted triangle_in signal : Outport
  wires:
  Sum4/1 -> sw/3
  modified triangle_shift/1 -> Sum4/1, Sum3/2, Sum2/2, Relational Operator6/2
  Switch3/1 -> sw/1
  Sum3/1 -> Switch3/3
  Sum2/1 -> Switch3/1
  sw/1 -> shifted triangle_in signal/1
  Relational Operator6/1 -> Switch3/2
  direction up/1 -> sw/2
  triangle_in/1 -> Relational Operator6/1, Sum3/1, Sum2/1, Sum4/2

== system IP_Core_SS_Switch_and_PWM/PWM_and_Switching_Signal_Control/GenPWM/Triangle shift1/Subsystem ==
  note: AND block replaced with
      | switches for better performance
  Zero_input : Inport
  converted triangle_shift : Inport  Port=2
  modified triangle_shift : Inport  Port=3
  triangle_in : Inport  Port=4
  direction down : Inport  Port=5
  Relational Operator11 : RelationalOperator  Operator=<=  OutDataTypeStr=boolean  RndMeth=Nearest
  Sum8 : Sum  Inputs=|-+
  Unary Minus : UnaryMinus
  and2_1 : Switch  Criteria=u2 > Threshold
  and2_2 : Switch  Criteria=u2 > Threshold
  shifted triangle_in signal : Outport
  enable_out : Outport  Port=2
  wires:
  direction down/1 -> and2_2/2
  Zero_input/1 -> and2_1/3, and2_2/3
  Relational Operator11/1 -> and2_1/2
  and2_1/1 -> and2_2/1
  Sum8/1 -> shifted triangle_in signal/1
  Unary Minus/1 -> Sum8/2, Relational Operator11/2
  triangle_in/1 -> Sum8/1, Relational Operator11/1
  converted triangle_shift/1 -> and2_1/1
  and2_2/1 -> enable_out/1
  modified triangle_shift/1 -> Unary Minus/1

== system IP_Core_SS_Switch_and_PWM/PWM_and_Switching_Signal_Control/GenPWM/Triangle shift1/Subsystem1 ==
  note: AND block replaced with
      | switches for better performance
  note: AND block replaced with
      | switches for better performance
  standardized peak of triangle : Inport
  triangle_in : Inport  Port=2
  converted triangle_shift : Inport  Port=3
  modified triangle_shift : Inport  Port=4
  Zero_input : Inport  Port=5
  direction up : Inport  Port=6
  Relational Operator2 : RelationalOperator  OutDataTypeStr=boolean  RndMeth=Nearest
  Sum11 : Sum  Inputs=++-  OutDataTypeStr=fixdt(1,21,17)
  Sum6 : Sum  Inputs=++|
  and1_1 : Switch  Criteria=u2 > Threshold
  and1_2 : Switch  Criteria=u2 > Threshold
  shifted triangle_in signal : Outport
  enable_out : Outport  Port=2
  wires:
  Sum11/1 -> shifted triangle_in signal/1
  Sum6/1 -> Relational Operator2/2, Sum11/2
  and1_1/1 -> and1_2/1
  Relational Operator2/1 -> and1_1/2
  Zero_input/1 -> and1_2/3, and1_1/3
  standardized peak of triangle/1 -> Sum6/2, Sum11/1
  and1_2/1 -> enable_out/1
  converted triangle_shift/1 -> and1_1/1
  direction up/1 -> and1_2/2
  triangle_in/1 -> Relational Operator2/1, Sum11/3
  modified triangle_shift/1 -> Sum6/1

== system IP_Core_SS_Switch_and_PWM/PWM_and_Switching_Signal_Control/GenPWM/Triangle shift1/Subsystem2 ==
  triangle_in : Inport
  modified triangle_shift : Inport  Port=2
  standardized peak of triangle : Inport  Port=3
  Zero_input : Inport  Port=4
  direction down : Inport  Port=5
  Relational Operator9 : RelationalOperator  OutDataTypeStr=boolean  RndMeth=Nearest
  Sum1 : Sum  Inputs=|-+
  Sum5 : Sum  Inputs=++-  OutDataTypeStr=fixdt(1,21,17)
  and : Switch  Criteria=u2 > Threshold
  shifted triangle_in signal : Outport
  enable_out : Outport  Port=2
  wires:
  standardized peak of triangle/1 -> Sum1/2, Sum5/2
  Zero_input/1 -> and/3
  Sum1/1 -> Relational Operator9/2, Sum5/1
  Relational Operator9/1 -> and/1
  direction down/1 -> and/2
  and/1 -> enable_out/1
  triangle_in/1 -> Relational Operator9/1, Sum5/3
  Sum5/1 -> shifted triangle_in signal/1
  modified triangle_shift/1 -> Sum1/1

== system IP_Core_SS_Switch_and_PWM/PWM_and_Switching_Signal_Control/GenPWM/Triangle shift1/Subsystem3 ==
  triangle_in : Inport
  modified triangle_shift : Inport  Port=2
  direction up : Inport  Port=3
  Relational Operator6 : RelationalOperator  Operator=<=  OutDataTypeStr=boolean  RndMeth=Nearest
  Sum2 : Sum  Inputs=|-+
  Sum3 : Sum  Inputs=|+-
  Sum4 : Sum  Inputs=|++
  Switch3 : Switch  Criteria=u2 > Threshold
  sw : Switch  Criteria=u2 > Threshold
  shifted triangle_in signal : Outport
  wires:
  Sum4/1 -> sw/3
  modified triangle_shift/1 -> Sum4/1, Sum3/2, Sum2/2, Relational Operator6/2
  Switch3/1 -> sw/1
  Sum3/1 -> Switch3/3
  Sum2/1 -> Switch3/1
  sw/1 -> shifted triangle_in signal/1
  Relational Operator6/1 -> Switch3/2
  direction up/1 -> sw/2
  triangle_in/1 -> Relational Operator6/1, Sum3/1, Sum2/1, Sum4/2

== system IP_Core_SS_Switch_and_PWM/PWM_and_Switching_Signal_Control/GenPWM/Triangle shift2/Subsystem ==
  note: AND block replaced with
      | switches for better performance
  Zero_input : Inport
  converted triangle_shift : Inport  Port=2
  modified triangle_shift : Inport  Port=3
  triangle_in : Inport  Port=4
  direction down : Inport  Port=5
  Relational Operator11 : RelationalOperator  Operator=<=  OutDataTypeStr=boolean  RndMeth=Nearest
  Sum8 : Sum  Inputs=|-+
  Unary Minus : UnaryMinus
  and2_1 : Switch  Criteria=u2 > Threshold
  and2_2 : Switch  Criteria=u2 > Threshold
  shifted triangle_in signal : Outport
  enable_out : Outport  Port=2
  wires:
  direction down/1 -> and2_2/2
  Zero_input/1 -> and2_1/3, and2_2/3
  Relational Operator11/1 -> and2_1/2
  and2_1/1 -> and2_2/1
  Sum8/1 -> shifted triangle_in signal/1
  Unary Minus/1 -> Sum8/2, Relational Operator11/2
  triangle_in/1 -> Sum8/1, Relational Operator11/1
  converted triangle_shift/1 -> and2_1/1
  and2_2/1 -> enable_out/1
  modified triangle_shift/1 -> Unary Minus/1

== system IP_Core_SS_Switch_and_PWM/PWM_and_Switching_Signal_Control/GenPWM/Triangle shift2/Subsystem1 ==
  note: AND block replaced with
      | switches for better performance
  note: AND block replaced with
      | switches for better performance
  standardized peak of triangle : Inport
  triangle_in : Inport  Port=2
  converted triangle_shift : Inport  Port=3
  modified triangle_shift : Inport  Port=4
  Zero_input : Inport  Port=5
  direction up : Inport  Port=6
  Relational Operator2 : RelationalOperator  OutDataTypeStr=boolean  RndMeth=Nearest
  Sum11 : Sum  Inputs=++-  OutDataTypeStr=fixdt(1,21,17)
  Sum6 : Sum  Inputs=++|
  and1_1 : Switch  Criteria=u2 > Threshold
  and1_2 : Switch  Criteria=u2 > Threshold
  shifted triangle_in signal : Outport
  enable_out : Outport  Port=2
  wires:
  Sum11/1 -> shifted triangle_in signal/1
  Sum6/1 -> Relational Operator2/2, Sum11/2
  and1_1/1 -> and1_2/1
  Relational Operator2/1 -> and1_1/2
  Zero_input/1 -> and1_2/3, and1_1/3
  standardized peak of triangle/1 -> Sum6/2, Sum11/1
  and1_2/1 -> enable_out/1
  converted triangle_shift/1 -> and1_1/1
  direction up/1 -> and1_2/2
  triangle_in/1 -> Relational Operator2/1, Sum11/3
  modified triangle_shift/1 -> Sum6/1

== system IP_Core_SS_Switch_and_PWM/PWM_and_Switching_Signal_Control/GenPWM/Triangle shift2/Subsystem2 ==
  triangle_in : Inport
  modified triangle_shift : Inport  Port=2
  standardized peak of triangle : Inport  Port=3
  Zero_input : Inport  Port=4
  direction down : Inport  Port=5
  Relational Operator9 : RelationalOperator  OutDataTypeStr=boolean  RndMeth=Nearest
  Sum1 : Sum  Inputs=|-+
  Sum5 : Sum  Inputs=++-  OutDataTypeStr=fixdt(1,21,17)
  and : Switch  Criteria=u2 > Threshold
  shifted triangle_in signal : Outport
  enable_out : Outport  Port=2
  wires:
  standardized peak of triangle/1 -> Sum1/2, Sum5/2
  Zero_input/1 -> and/3
  Sum1/1 -> Relational Operator9/2, Sum5/1
  Relational Operator9/1 -> and/1
  direction down/1 -> and/2
  and/1 -> enable_out/1
  triangle_in/1 -> Relational Operator9/1, Sum5/3
  Sum5/1 -> shifted triangle_in signal/1
  modified triangle_shift/1 -> Sum1/1

== system IP_Core_SS_Switch_and_PWM/PWM_and_Switching_Signal_Control/GenPWM/Triangle shift2/Subsystem3 ==
  triangle_in : Inport
  modified triangle_shift : Inport  Port=2
  direction up : Inport  Port=3
  Relational Operator6 : RelationalOperator  Operator=<=  OutDataTypeStr=boolean  RndMeth=Nearest
  Sum2 : Sum  Inputs=|-+
  Sum3 : Sum  Inputs=|+-
  Sum4 : Sum  Inputs=|++
  Switch3 : Switch  Criteria=u2 > Threshold
  sw : Switch  Criteria=u2 > Threshold
  shifted triangle_in signal : Outport
  wires:
  Sum4/1 -> sw/3
  modified triangle_shift/1 -> Sum4/1, Sum3/2, Sum2/2, Relational Operator6/2
  Switch3/1 -> sw/1
  Sum3/1 -> Switch3/3
  Sum2/1 -> Switch3/1
  sw/1 -> shifted triangle_in signal/1
  Relational Operator6/1 -> Switch3/2
  direction up/1 -> sw/2
  triangle_in/1 -> Relational Operator6/1, Sum3/1, Sum2/1, Sum4/2

== system IP_Core_SS_Switch_and_PWM/PWM_and_Switching_Signal_Control1/GenPWM/Triangle shift/Subsystem ==
  note: AND block replaced with
      | switches for better performance
  Zero_input : Inport
  converted triangle_shift : Inport  Port=2
  modified triangle_shift : Inport  Port=3
  triangle_in : Inport  Port=4
  direction down : Inport  Port=5
  Relational Operator11 : RelationalOperator  Operator=<=  OutDataTypeStr=boolean  RndMeth=Nearest
  Sum8 : Sum  Inputs=|-+
  Unary Minus : UnaryMinus
  and2_1 : Switch  Criteria=u2 > Threshold
  and2_2 : Switch  Criteria=u2 > Threshold
  shifted triangle_in signal : Outport
  enable_out : Outport  Port=2
  wires:
  direction down/1 -> and2_2/2
  Zero_input/1 -> and2_1/3, and2_2/3
  Relational Operator11/1 -> and2_1/2
  and2_1/1 -> and2_2/1
  Sum8/1 -> shifted triangle_in signal/1
  Unary Minus/1 -> Sum8/2, Relational Operator11/2
  triangle_in/1 -> Sum8/1, Relational Operator11/1
  converted triangle_shift/1 -> and2_1/1
  and2_2/1 -> enable_out/1
  modified triangle_shift/1 -> Unary Minus/1

== system IP_Core_SS_Switch_and_PWM/PWM_and_Switching_Signal_Control1/GenPWM/Triangle shift/Subsystem1 ==
  note: AND block replaced with
      | switches for better performance
  note: AND block replaced with
      | switches for better performance
  standardized peak of triangle : Inport
  triangle_in : Inport  Port=2
  converted triangle_shift : Inport  Port=3
  modified triangle_shift : Inport  Port=4
  Zero_input : Inport  Port=5
  direction up : Inport  Port=6
  Relational Operator2 : RelationalOperator  OutDataTypeStr=boolean  RndMeth=Nearest
  Sum11 : Sum  Inputs=++-  OutDataTypeStr=fixdt(1,21,17)
  Sum6 : Sum  Inputs=++|
  and1_1 : Switch  Criteria=u2 > Threshold
  and1_2 : Switch  Criteria=u2 > Threshold
  shifted triangle_in signal : Outport
  enable_out : Outport  Port=2
  wires:
  Sum11/1 -> shifted triangle_in signal/1
  Sum6/1 -> Relational Operator2/2, Sum11/2
  and1_1/1 -> and1_2/1
  Relational Operator2/1 -> and1_1/2
  Zero_input/1 -> and1_2/3, and1_1/3
  standardized peak of triangle/1 -> Sum6/2, Sum11/1
  and1_2/1 -> enable_out/1
  converted triangle_shift/1 -> and1_1/1
  direction up/1 -> and1_2/2
  triangle_in/1 -> Relational Operator2/1, Sum11/3
  modified triangle_shift/1 -> Sum6/1

== system IP_Core_SS_Switch_and_PWM/PWM_and_Switching_Signal_Control1/GenPWM/Triangle shift/Subsystem2 ==
  triangle_in : Inport
  modified triangle_shift : Inport  Port=2
  standardized peak of triangle : Inport  Port=3
  Zero_input : Inport  Port=4
  direction down : Inport  Port=5
  Relational Operator9 : RelationalOperator  OutDataTypeStr=boolean  RndMeth=Nearest
  Sum1 : Sum  Inputs=|-+
  Sum5 : Sum  Inputs=++-  OutDataTypeStr=fixdt(1,21,17)
  and : Switch  Criteria=u2 > Threshold
  shifted triangle_in signal : Outport
  enable_out : Outport  Port=2
  wires:
  standardized peak of triangle/1 -> Sum1/2, Sum5/2
  Zero_input/1 -> and/3
  Sum1/1 -> Relational Operator9/2, Sum5/1
  Relational Operator9/1 -> and/1
  direction down/1 -> and/2
  and/1 -> enable_out/1
  triangle_in/1 -> Relational Operator9/1, Sum5/3
  Sum5/1 -> shifted triangle_in signal/1
  modified triangle_shift/1 -> Sum1/1

== system IP_Core_SS_Switch_and_PWM/PWM_and_Switching_Signal_Control1/GenPWM/Triangle shift/Subsystem3 ==
  triangle_in : Inport
  modified triangle_shift : Inport  Port=2
  direction up : Inport  Port=3
  Relational Operator6 : RelationalOperator  Operator=<=  OutDataTypeStr=boolean  RndMeth=Nearest
  Sum2 : Sum  Inputs=|-+
  Sum3 : Sum  Inputs=|+-
  Sum4 : Sum  Inputs=|++
  Switch3 : Switch  Criteria=u2 > Threshold
  sw : Switch  Criteria=u2 > Threshold
  shifted triangle_in signal : Outport
  wires:
  Sum4/1 -> sw/3
  modified triangle_shift/1 -> Sum4/1, Sum3/2, Sum2/2, Relational Operator6/2
  Switch3/1 -> sw/1
  Sum3/1 -> Switch3/3
  Sum2/1 -> Switch3/1
  sw/1 -> shifted triangle_in signal/1
  Relational Operator6/1 -> Switch3/2
  direction up/1 -> sw/2
  triangle_in/1 -> Relational Operator6/1, Sum3/1, Sum2/1, Sum4/2

== system IP_Core_SS_Switch_and_PWM/PWM_and_Switching_Signal_Control1/GenPWM/Triangle shift1/Subsystem ==
  note: AND block replaced with
      | switches for better performance
  Zero_input : Inport
  converted triangle_shift : Inport  Port=2
  modified triangle_shift : Inport  Port=3
  triangle_in : Inport  Port=4
  direction down : Inport  Port=5
  Relational Operator11 : RelationalOperator  Operator=<=  OutDataTypeStr=boolean  RndMeth=Nearest
  Sum8 : Sum  Inputs=|-+
  Unary Minus : UnaryMinus
  and2_1 : Switch  Criteria=u2 > Threshold
  and2_2 : Switch  Criteria=u2 > Threshold
  shifted triangle_in signal : Outport
  enable_out : Outport  Port=2
  wires:
  direction down/1 -> and2_2/2
  Zero_input/1 -> and2_1/3, and2_2/3
  Relational Operator11/1 -> and2_1/2
  and2_1/1 -> and2_2/1
  Sum8/1 -> shifted triangle_in signal/1
  Unary Minus/1 -> Sum8/2, Relational Operator11/2
  triangle_in/1 -> Sum8/1, Relational Operator11/1
  converted triangle_shift/1 -> and2_1/1
  and2_2/1 -> enable_out/1
  modified triangle_shift/1 -> Unary Minus/1

== system IP_Core_SS_Switch_and_PWM/PWM_and_Switching_Signal_Control1/GenPWM/Triangle shift1/Subsystem1 ==
  note: AND block replaced with
      | switches for better performance
  note: AND block replaced with
      | switches for better performance
  standardized peak of triangle : Inport
  triangle_in : Inport  Port=2
  converted triangle_shift : Inport  Port=3
  modified triangle_shift : Inport  Port=4
  Zero_input : Inport  Port=5
  direction up : Inport  Port=6
  Relational Operator2 : RelationalOperator  OutDataTypeStr=boolean  RndMeth=Nearest
  Sum11 : Sum  Inputs=++-  OutDataTypeStr=fixdt(1,21,17)
  Sum6 : Sum  Inputs=++|
  and1_1 : Switch  Criteria=u2 > Threshold
  and1_2 : Switch  Criteria=u2 > Threshold
  shifted triangle_in signal : Outport
  enable_out : Outport  Port=2
  wires:
  Sum11/1 -> shifted triangle_in signal/1
  Sum6/1 -> Relational Operator2/2, Sum11/2
  and1_1/1 -> and1_2/1
  Relational Operator2/1 -> and1_1/2
  Zero_input/1 -> and1_2/3, and1_1/3
  standardized peak of triangle/1 -> Sum6/2, Sum11/1
  and1_2/1 -> enable_out/1
  converted triangle_shift/1 -> and1_1/1
  direction up/1 -> and1_2/2
  triangle_in/1 -> Relational Operator2/1, Sum11/3
  modified triangle_shift/1 -> Sum6/1

== system IP_Core_SS_Switch_and_PWM/PWM_and_Switching_Signal_Control1/GenPWM/Triangle shift1/Subsystem2 ==
  triangle_in : Inport
  modified triangle_shift : Inport  Port=2
  standardized peak of triangle : Inport  Port=3
  Zero_input : Inport  Port=4
  direction down : Inport  Port=5
  Relational Operator9 : RelationalOperator  OutDataTypeStr=boolean  RndMeth=Nearest
  Sum1 : Sum  Inputs=|-+
  Sum5 : Sum  Inputs=++-  OutDataTypeStr=fixdt(1,21,17)
  and : Switch  Criteria=u2 > Threshold
  shifted triangle_in signal : Outport
  enable_out : Outport  Port=2
  wires:
  standardized peak of triangle/1 -> Sum1/2, Sum5/2
  Zero_input/1 -> and/3
  Sum1/1 -> Relational Operator9/2, Sum5/1
  Relational Operator9/1 -> and/1
  direction down/1 -> and/2
  and/1 -> enable_out/1
  triangle_in/1 -> Relational Operator9/1, Sum5/3
  Sum5/1 -> shifted triangle_in signal/1
  modified triangle_shift/1 -> Sum1/1
